simulink model "coursehold"  (R2017a)
settings: Solver=VariableStepAuto  StartTime=0.0  StopTime=50  RelTol=1e-3
undefined symbols (not defined in the file): a_phi1, a_phi2, delta_a_max, P
settings Model: Creator=pizzaslayer  LastModifiedBy=Parth

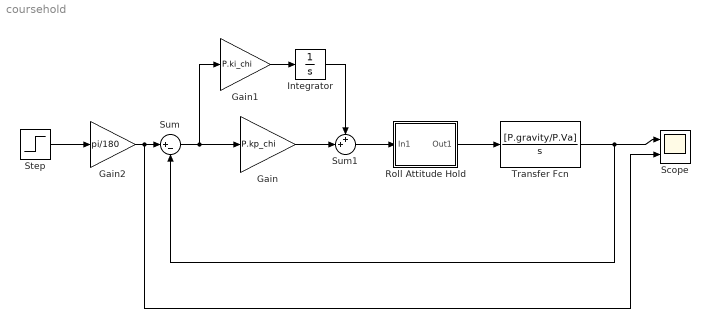
== system coursehold ==
  Gain : Gain  Gain=P.kp_chi
  Gain1 : Gain  Gain=P.ki_chi
  Gain2 : Gain  Gain=pi/180
  Integrator : Integrator
  "Roll Attitude Hold " : Subsystem
  Scope : Scope  NumInputPorts=2
  Step : Step  Time=0  After=25  SampleTime=0
  Sum : Sum  Inputs=|+-
  Sum1 : Sum  Inputs=++|
  Transfer Fcn : TransferFcn  Numerator=[P.gravity/P.Va]  Denominator=[1 0]
  wires:
  Sum1/1 -> "Roll Attitude Hold "/1(In1)
  Sum/1 -> Gain/1, Gain1/1
  Gain1/1 -> Integrator/1
  Integrator/1 -> Sum1/1
  Gain/1 -> Sum1/2
  "Roll Attitude Hold "/1(Out1) -> Transfer Fcn/1
  Transfer Fcn/1 -> Scope/1, Sum/2
  Step/1 -> Gain2/1
  Gain2/1 -> Scope/2, Sum/1

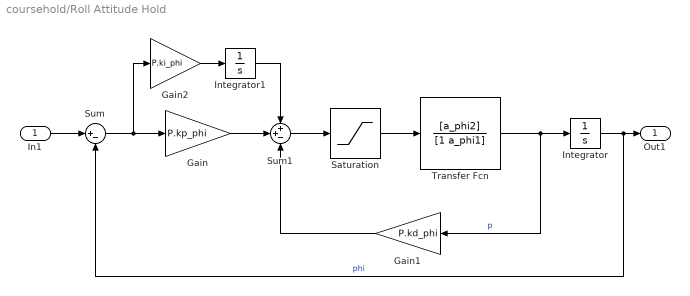
== system coursehold/Roll Attitude Hold  ==
  In1 : Inport
  Gain : Gain  Gain=P.kp_phi
  Gain1 : Gain  Gain=P.kd_phi
  Gain2 : Gain  Gain=P.ki_phi
  Integrator : Integrator
  Integrator1 : Integrator
  Saturation : Saturate  UpperLimit=delta_a_max  LowerLimit=-delta_a_max
  Sum : Sum  Inputs=|+-
  Sum1 : Sum  Inputs=++-
  Transfer Fcn : TransferFcn  Numerator=[a_phi2]  Denominator=[1 a_phi1]
  Out1 : Outport
  wires:
  Integrator1/1 -> Sum1/1
  Saturation/1 -> Transfer Fcn/1
  Gain1/1 -> Sum1/3
  Sum/1 -> Gain2/1, Gain/1
  In1/1 -> Sum/1
  Gain2/1 -> Integrator1/1
  Integrator/1 -> Out1/1, Sum/2  "phi"
  Transfer Fcn/1 -> Gain1/1, Integrator/1  "p"
  Sum1/1 -> Saturation/1
  Gain/1 -> Sum1/2
